simulink model "NMPC_CSTR_R2017a"  (R2017a)
settings: Solver=VariableStepAuto  StartTime=0.0  StopTime=400  RelTol=1e-3
values from neighbouring files (symbols this model uses):
  Ts = 1    [NonlinearMPC_siso_CSTR.m]    (also in TITO_CSTR_StateFcnDT.m)
  u0 = 103.41    [NonlinearMPC_siso_CSTR.m]
undefined symbols (not defined in the file or in its folder): sigbuilder_block
libraries: mpclib x1, simulink x1
settings Model: Creator=CHEMENG  LastModifiedBy=USER
settings DataIOCC: ReturnWorkspaceOutputs=on
settings DebuggingCC: SFMachineParentedDataDiag=error
settings SFSimCC: SimUseLocalCustomCode=on
settings RTWCC: RTWUseLocalCustomCode=on

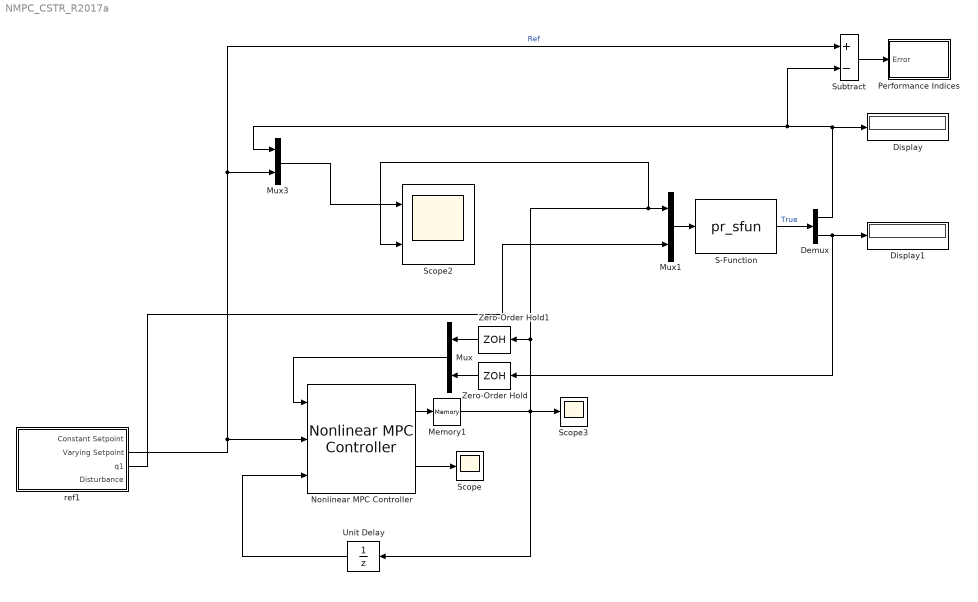
== system NMPC_CSTR_R2017a ==
  Demux : Demux  Outputs=2
  Display : Display
  Display1 : Display
  Memory1 : Memory  X0=103.41
  Mux : Mux  Inputs=2
  Mux1 : Mux  Inputs=2
  Mux3 : Mux  Inputs=2
  Nonlinear MPC Controller : mpclib/Nonlinear MPC Controller  SCDEnableBlockLinearizationSpecification=on  nlmpcobj=nlobj  UseObjectTs=on  UseMEX=off  md_enabled=off  mvtarget_enabled=off  param_enabled=off  cost_enabled=off  mvseq_enabled=off  stateseq_enabled=off  ovseq_enabled=off  slack_enabled=off  status_enabled=on  ov_min=off  ov_max=off  mv_min=off  mv_max=off  mvrate_min=off  mvrate_max=off  state_min=off  state_max=off  ov_weight=off  mv_weight=off  mvrate_weight=off  ecr_weight=off  nlp_initialize=off
  Performance Indices : Subsystem
  S-Function : S-Function  FunctionName=pr_sfun  SFunctionDeploymentMode=off  EnableBusSupport=off
  Scope : Scope
  Scope2 : Scope  NumInputPorts=2
  Scope3 : Scope
  Subtract : Sum  Inputs=+-
  Unit Delay : UnitDelay  InitialCondition=u0  SampleTime=-1  HasFrameUpgradeWarning=on
  Zero-Order Hold : ZeroOrderHold  SampleTime=Ts
  Zero-Order Hold1 : ZeroOrderHold  SampleTime=Ts
  "ref1 " : Subsystem  Tag=STV Subsys  LoadFcn=sigbuilder_block('load');  StartFcn=sigbuilder_block('start');  StopFcn=sigbuilder_block('stop');  ClipboardFcn=sigbuilder_block('clipboard');  mask(Sigbuilder block){tuvar=[0:10]}
      mask help: Simulink:masks:SigbuilderBlock_MD
      mask init:
      | if ~strcmp(get_param(bdroot(gcbh),'SimulationStatus'),'stopped') tuvar = sigbuilder_block('maskInit'); end
      settings: CopyFcn=sigbuilder_block('copy');  DeleteFcn=sigbuilder_block('delete');  ModelCloseFcn=sigbuilder_block('modelClose');  PreSaveFcn=sigbuilder_block('preSave');  PauseFcn=sigbuilder_block('pause');  ContinueFcn=sigbuilder_block('continue');  NameChangeFcn=sigbuilder_block('namechange');  OpenFcn=sigbuilder_block('open',[5.5 0 949 448 ]);  CloseFcn=sigbuilder_block('close');
      mask Display: plot(0, 0, 100, 100,[2, 2, 32, 32, 2], [68, 8, 8, 68, 68],[32, 2], [38, 38], [32, 19, 2],[53, 60, 44], [32, 17, 17, 2],[16, 16, 31, 31]);txt = getActiveGroup(gcbh);text(2, 100, txt,'verticalAlignment', 'top');
  wires:
  Unit Delay/1 -> Nonlinear MPC Controller/3
  Zero-Order Hold/1 -> Mux/2
  Zero-Order Hold1/1 -> Mux/1
  Demux/2 -> Display1/1, Zero-Order Hold/1
  Mux3/1 -> Scope2/1
  Nonlinear MPC Controller/2 -> Scope/1
  Mux1/1 -> S-Function/1
  "ref1 "/3(q1) -> Mux1/2
  S-Function/1 -> Demux/1  "True"
  Nonlinear MPC Controller/1 -> Memory1/1
  Memory1/1 -> Scope3/1, Mux1/1, Scope2/2, Zero-Order Hold1/1, Unit Delay/1
  Mux/1 -> Nonlinear MPC Controller/1
  "ref1 "/2(Varying Setpoint) -> Subtract/1, Mux3/2, Nonlinear MPC Controller/2  "Ref"
  Subtract/1 -> Performance Indices/1(Error)
  Demux/1 -> Subtract/2, Mux3/1, Display/1

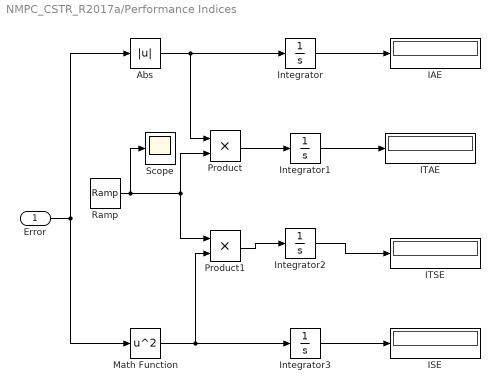
== system NMPC_CSTR_R2017a/Performance Indices ==
  Error : Inport
  Abs : Abs
  IAE : Display
  ISE : Display
  ITAE : Display
  ITSE : Display
  Integrator{,1..3} (4 alike) : Integrator
  Math Function : Math  Operator=square  SaturateOnIntegerOverflow=on
  Product : Product  RndMeth=Zero
  Product1 : Product  RndMeth=Zero
  Ramp : simulink/Sources/Ramp  slope=1  start=0  X0=0
  Scope : Scope
  wires:
  Error/1 -> Math Function/1, Abs/1
  Abs/1 -> Integrator/1, Product/1
  Integrator/1 -> IAE/1
  Ramp/1 -> Product/2, Product1/1, Scope/1
  Math Function/1 -> Integrator3/1, Product1/2
  Product1/1 -> Integrator2/1
  Product/1 -> Integrator1/1
  Integrator3/1 -> ISE/1
  Integrator2/1 -> ITSE/1
  Integrator1/1 -> ITAE/1

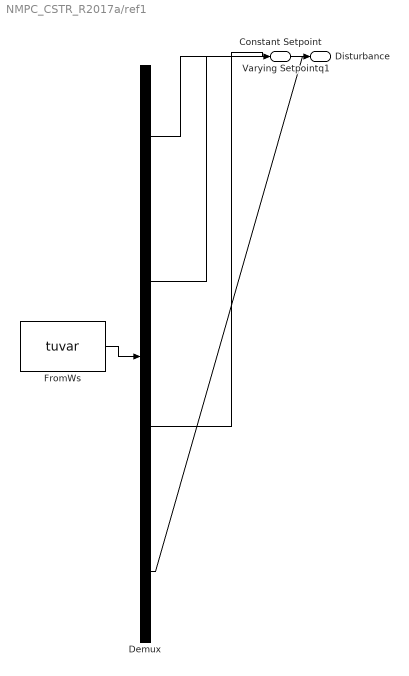
== system NMPC_CSTR_R2017a/ref1  ==
  Demux : Demux  Tag=STV Demux
      settings: DisplayOption=none
  FromWs : FromWorkspace  Tag=STV FromWs  VariableName=tuvar
      SigBuilderData=|
      | common.afterFinalStr = 'Extrapolate'
      | common.sampleTime = 0
      | dataSet.timeRange = [0 400]
      | dataSet.name = 'Group 1'
      | sbobj.Groups.Name = 'Group 1'
      | sbobj.Groups.Signals(1).Name = 'Constant Setpoint'
      | sbobj.Groups.Signals(1).XData = [0 400]
      | sbobj.Groups.Signals(1).YData = [0.1 0.1]
      | sbobj.Groups.Signals(2).Name = 'Varying Setpoint'
      | sbobj.Groups.Signals(2).XData = [0 50 50 150 150 300 300 400]
      | sbobj.Groups.Signals(2).YData = [0.085 0.085 0.1 0.1 0.04 0.04 0.1 0.1]
      | sbobj.Groups.Signals(3).Name = 'q1'
      | sbobj.Groups.Signals(3).XData = [0 400]
      | sbobj.Groups.Signals(3).YData = [100 100]
      | sbobj.Groups.Signals(4).Name = 'Disturbance'
      | sbobj.Groups.Signals(4).XData = [0 50 50 150 150 300 300 400]
      | sbobj.Groups.Signals(4).YData = [100 100 95 95 105 105 100 100]
      | sbobj.Groups.TimeRange = [0 400]
  Constant Setpoint : Outport  Tag=STV Outport
  Varying Setpoint : Outport  Tag=STV Outport  Port=2
  q1 : Outport  Tag=STV Outport  Port=3
  Disturbance : Outport  Tag=STV Outport  Port=4
  wires:
  FromWs/1 -> Demux/1
  Demux/1 -> Constant Setpoint/1
  Demux/2 -> Varying Setpoint/1
  Demux/3 -> q1/1
  Demux/4 -> Disturbance/1
